simulink model "SimulinkNewUpdate"  (R2025a)
settings: Solver=VariableStepAuto  StartTime=0.0  StopTime=10.0  RelTol=1e-3
values from neighbouring files (symbols this model uses):
  AUM = 3.057    [Parameter.m]
  g = -9.8    [Parameter.m]
  H = 0.05    [Parameter.m]
  L = 0.25    [Parameter.m]
  rho = 1.18195    [Parameter.m]
  W = diag([0.994, 0.003, 0.003, 0.994, 0.003, 0.003,            0.994, 0.003, 0.003, 0.994, 0.003, 0.003])    [Parameter.m]
libraries: slpidlib x10, matrix_library x8, robotcorelib x4, simulink x1, uavalgslib x1, aerolibobsolete x1
(part 2 of 2)

== system SimulinkNewUpdate/Subsystem2/velocity control ==
  CmdvDown : Inport
  In Bus Element1 : Inport  Port=2  PortName=sensor
  In Bus Element : Inport  Port=2  PortName=sensor  Element=vZBody
  Discrete PID Controller : slpidlib/PID Controller  Controller=PID  Form=Parallel  TimeDomain=Discrete-time  UseExternalTs=off  SampleTime=0.005  IntegratorMethod=Forward Euler  FilterMethod=Forward Euler  ControllerParametersSource=external  P=1  I=1  UseKiTs=off  D=0  UseExternalDerivativeSource=off  N=100  UseFilter=on  TunerSelectOption=Transfer Function Based (PID Tuner App)  InitialConditionSource=external  InitialConditionForIntegrator=0  InitialConditionForFilter=0  DifferentiatorICPrevScaledInput=0  ExternalReset=none  TrackingMode=off  Kt=1  LimitOutput=on  SatLimitsSource=internal  UpperSaturationLimit=inf  LowerSaturationLimit=-inf  LinearizeAsGain=off  AntiWindupMode=none  Kb=1  LimitIntegrator=off  UpperIntegratorSaturationLimit=inf  LowerIntegratorSaturationLimit=-inf  POutMin=[]  POutMax=[]  IOutMin=[]  IOutMax=[]  DOutMin=[]  DOutMax=[]  NOutMin=[]  NOutMax=[]  SumOutMin=[]  SumOutMax=[]  SaturationOutMin=[]  SaturationOutMax=[]  PParamMin=[]  PParamMax=[]  IParamMin=[]  IParamMax=[]  DParamMin=[]  DParamMax=[]  NParamMin=[]  NParamMax=[]  KbParamMin=[]  KbParamMax=[]  KtParamMin=[]  KtParamMax=[]  KbOutMin=[]  KbOutMax=[]  KtOutMin=[]  KtOutMax=[]  IntegratorOutMin=[]  IntegratorOutMax=[]  FilterOutMin=[]  FilterOutMax=[]  SumI1OutMin=[]  SumI1OutMax=[]  SumI2OutMin=[]  SumI2OutMax=[]  SumI3OutMin=[]  SumI3OutMax=[]  SumI4OutMin=[]  SumI4OutMax=[]  SumDOutMin=[]  SumDOutMax=[]  DifferentiatorOutMin=[]  DifferentiatorOutMax=[]  FilterDiffOutCoefMin=[]  FilterDiffOutCoefMax=[]  ReciprocalOutMin=[]  ReciprocalOutMax=[]  SumDenOutMin=[]  SumDenOutMax=[]  SumNumOutMin=[]  SumNumOutMax=[]  DivideOutMin=[]  DivideOutMax=[]  UdiffTsProdOutMin=[]  UdiffTsProdOutMax=[]  NTsProdOutMin=[]  NTsProdOutMax=[]  UintegralTsProdOutMin=[]  UintegralTsProdOutMax=[]  UngainTsProdOutMin=[]  UngainTsProdOutMax=[]  ClampingZeroOutDataTypeStr=Inherit: Inherit via back propagation  ClampingZeroOutMin=[]  ClampingZeroOutMax=[]  FilterDenConstantOutDataTypeStr=Inherit: Inherit via back propagation  FilterDenConstantOutMin=[]  FilterDenConstantOutMax=[]  PCopyOutDataTypeStr=Inherit: Inherit via back propagation  PCopyOutMin=[]  PCopyOutMax=[]  NCopyOutDataTypeStr=Inherit: Inherit via back propagation  NCopyOutMin=[]  NCopyOutMax=[]  IntegratorContinuousStateAttributes=''  IntegratorStateMustResolveToSignalObject=off  IntegratorRTWStateStorageClass=Auto  FilterContinuousStateAttributes=''  FilterStateMustResolveToSignalObject=off  FilterRTWStateStorageClass=Auto  ParallelPVariant=ExternalParameters  IdealPVariant=Disabled  IVariant=ExternalParameters  DVariant=ExternalParameters  IntegratorVariant=Discrete  SatVariant=Enabled  AWVariant=Passthrough  PCopyVariant=Disabled  TRVariant=Disabled  FdbkBlocksVariant=Forward  IdealPFdbkVariant=Disabled  SatFdbkVariant=Disabled  DerivativeFilterVariant=ForwardEulerFilter  NVariant=ExternalParameters  NCopyVariant=Disabled  FilterICVariant=ExternalICs  IntegratorICVariant=ExternalICs  ExternalResetVariant=Disabled  TRSumVariant=Passthrough  SumFdbkVariant=Disabled  SumVariant=Sum_PID  TsampFilterVariant=InternalTs  TsampNgainVariant=Passthrough  TsampIntegralVariant=Disabled_SignalSpec  ExternalSaturationOutDataTypeStr=Inherit: Same as second input  DerivativeSourceVariant=ErrorSignal  PreIntVariant=InternalPreInt
      settings: LibrarySourceBlock=simulink/Discrete/Discrete PID Controller
  Gain : Gain  Gain=1000
  Kd : Constant
  Ki : Constant
  Kp : Constant
  N : Constant
  N1 : Constant
  N2 : Constant
  Roll and Pitch compensation : Subsystem
  Sum : Sum  Inputs=|+-
  cmdThrust : Outport
  wires:
  CmdvDown/1 -> Sum/1
  Sum/1 -> Discrete PID Controller/1
  Kp/1 -> Discrete PID Controller/2
  Ki/1 -> Discrete PID Controller/3
  Kd/1 -> Discrete PID Controller/4
  N/1 -> Discrete PID Controller/5
  Discrete PID Controller/1 -> Gain/1
  N1/1 -> Discrete PID Controller/6
  N2/1 -> Discrete PID Controller/7
  Gain/1 -> Roll and Pitch compensation/1(thrust)
  Roll and Pitch compensation/1(thrustCompensation) -> cmdThrust/1
  In Bus Element1/1 -> Roll and Pitch compensation/2(sensing)
  In Bus Element/1 -> Sum/2

== system SimulinkNewUpdate/Vehicle Dynamic1/Subsystem1 ==
  omega : Inport
  Bus Creator : BusCreator  Inputs=3
  Demux : Demux  Outputs=3
  Rotation : Outport
  wires:
  omega/1 -> Demux/1
  Bus Creator/1 -> Rotation/1
  Demux/1 -> Bus Creator/1  "p"
  Demux/2 -> Bus Creator/2  "q"
  Demux/3 -> Bus Creator/3  "r"

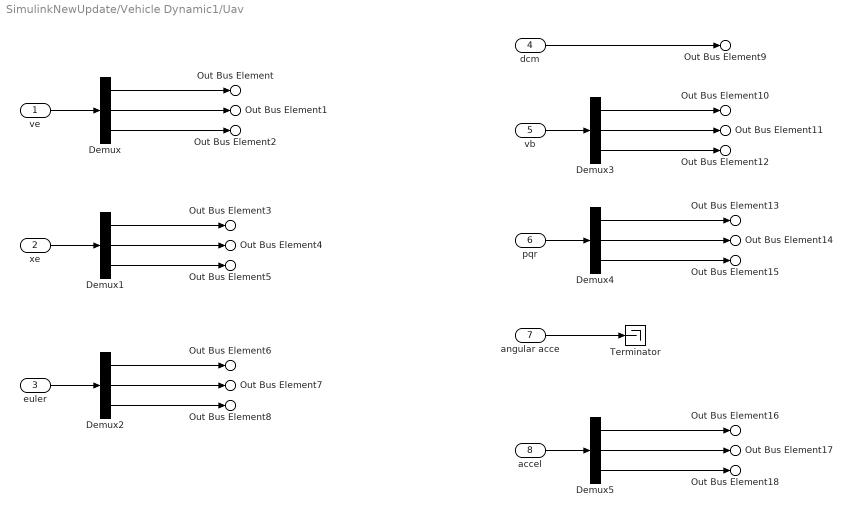
== system SimulinkNewUpdate/Vehicle Dynamic1/Uav ==
  ve : Inport
  xe : Inport  Port=2
  euler : Inport  Port=3
  dcm : Inport  Port=4
  vb : Inport  Port=5
  pqr : Inport  Port=6
  angular acce : Inport  Port=7
  accel : Inport  Port=8
  Demux{,1..5} (6 alike) : Demux  Outputs=3
  Terminator : Terminator
  Out Bus Element9 : Outport  PortName=UavState  Element=DCM
  Out Bus Element6 : Outport  PortName=UavState  Element=roll
  Out Bus Element7 : Outport  PortName=UavState  Element=pitch
  Out Bus Element8 : Outport  PortName=UavState  Element=yaw
  Out Bus Element : Outport  PortName=UavState  Element=veX
  Out Bus Element1 : Outport  PortName=UavState  Element=veY
  Out Bus Element2 : Outport  PortName=UavState  Element=veZ
  Out Bus Element3 : Outport  PortName=UavState  Element=x
  Out Bus Element4 : Outport  PortName=UavState  Element=y
  Out Bus Element5 : Outport  PortName=UavState  Element=z
  Out Bus Element10 : Outport  PortName=UavState  Element=vXBody
  Out Bus Element11 : Outport  PortName=UavState  Element=vYBody
  Out Bus Element12 : Outport  PortName=UavState  Element=vZBody
  Out Bus Element13 : Outport  PortName=UavState  Element=wx
  Out Bus Element14 : Outport  PortName=UavState  Element=wy
  Out Bus Element15 : Outport  PortName=UavState  Element=wz
  Out Bus Element16 : Outport  PortName=UavState  Element=accXBody
  Out Bus Element17 : Outport  PortName=UavState  Element=accYBody
  Out Bus Element18 : Outport  PortName=UavState  Element=accZBody
  wires:
  ve/1 -> Demux/1
  Demux/1 -> Out Bus Element/1
  Demux/2 -> Out Bus Element1/1
  Demux/3 -> Out Bus Element2/1
  xe/1 -> Demux1/1
  Demux1/1 -> Out Bus Element3/1
  Demux1/2 -> Out Bus Element4/1
  Demux1/3 -> Out Bus Element5/1
  euler/1 -> Demux2/1
  Demux2/1 -> Out Bus Element6/1
  Demux2/2 -> Out Bus Element7/1
  Demux2/3 -> Out Bus Element8/1
  dcm/1 -> Out Bus Element9/1
  vb/1 -> Demux3/1
  Demux3/1 -> Out Bus Element10/1
  Demux3/2 -> Out Bus Element11/1
  Demux3/3 -> Out Bus Element12/1
  pqr/1 -> Demux4/1
  Demux4/1 -> Out Bus Element13/1
  Demux4/2 -> Out Bus Element14/1
  Demux4/3 -> Out Bus Element15/1
  angular acce/1 -> Terminator/1
  accel/1 -> Demux5/1
  Demux5/1 -> Out Bus Element16/1
  Demux5/2 -> Out Bus Element17/1
  Demux5/3 -> Out Bus Element18/1

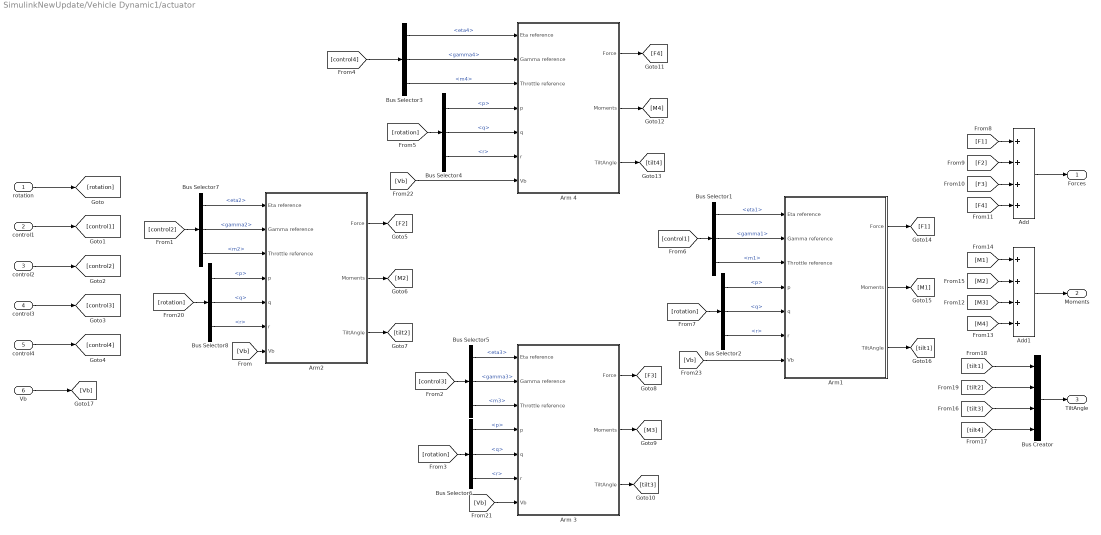
== system SimulinkNewUpdate/Vehicle Dynamic1/actuator ==
  rotation : Inport
  control1 : Inport  Port=2
  control2 : Inport  Port=3
  control3 : Inport  Port=4
  control4 : Inport  Port=5
  Vb : Inport  Port=6
  Add : Sum  Inputs=++++
  Add1 : Sum  Inputs=++++
  Arm 3 : Subsystem
  Arm 4 : Subsystem
  Arm1 : Subsystem
  Arm2 : Subsystem
  Bus Creator : BusCreator  Inputs=4
  Bus Selector1 : BusSelector  OutputSignals=eta1,gamma1,m1
  Bus Selector{2,4,6,8} (4 alike) : BusSelector  OutputSignals=p,q,r
  Bus Selector3 : BusSelector  OutputSignals=eta4,gamma4,m4
  Bus Selector5 : BusSelector  OutputSignals=eta3,gamma3,m3
  Bus Selector7 : BusSelector  OutputSignals=eta2,gamma2,m2
  Forces : Outport
  Moments : Outport  Port=2
  TiltAngle : Outport  Port=3
  wires:
  control3/1 -> [control3]
  Add/1 -> Forces/1
  [F4] -> Add/4
  [M3] -> Add1/3
  [control1] -> Bus Selector1/1
  Arm 4/1(Force) -> [F4]
  [M2] -> Add1/2
  Arm2/1(Force) -> [F2]
  [M1] -> Add1/1
  [M4] -> Add1/4
  Add1/1 -> Moments/1
  Arm 3/1(Force) -> [F3]
  Arm 4/2(Moments) -> [M4]
  Arm 3/2(Moments) -> [M3]
  control1/1 -> [control1]
  Arm2/3(TiltAngle) -> [tilt2]
  Arm 3/3(TiltAngle) -> [tilt3]
  control2/1 -> [control2]
  Arm2/2(Moments) -> [M2]
  Arm 4/3(TiltAngle) -> [tilt4]
  rotation/1 -> [rotation]
  control4/1 -> [control4]
  [F3] -> Add/3
  [F1] -> Add/1
  [F2] -> Add/2
  [tilt1] -> Bus Creator/1
  [tilt2] -> Bus Creator/2
  [tilt3] -> Bus Creator/3
  [tilt4] -> Bus Creator/4
  Bus Creator/1 -> TiltAngle/1
  [rotation] -> Bus Selector2/1
  Bus Selector1/1 -> Arm1/1(Eta reference)  "<eta1>"
  Bus Selector1/2 -> Arm1/2(Gamma reference)  "<gamma1>"
  Bus Selector1/3 -> Arm1/3(Throttle reference)  "<m1>"
  [control4] -> Bus Selector3/1
  [control3] -> Bus Selector5/1
  [control2] -> Bus Selector7/1
  Bus Selector5/1 -> Arm 3/1(Eta reference)  "<eta3>"
  Bus Selector5/2 -> Arm 3/2(Gamma reference)  "<gamma3>"
  Bus Selector5/3 -> Arm 3/3(Throttle reference)  "<m3>"
  Bus Selector7/1 -> Arm2/1(Eta reference)  "<eta2>"
  Bus Selector7/2 -> Arm2/2(Gamma reference)  "<gamma2>"
  Bus Selector7/3 -> Arm2/3(Throttle reference)  "<m2>"
  Bus Selector6/1 -> Arm 3/4(p)  "<p>"
  [rotation] -> Bus Selector6/1
  [rotation] -> Bus Selector8/1
  [rotation] -> Bus Selector4/1
  Bus Selector6/2 -> Arm 3/5(q)  "<q>"
  Bus Selector6/3 -> Arm 3/6(r)  "<r>"
  Arm1/1(Force) -> [F1]
  Arm1/2(Moments) -> [M1]
  Arm1/3(TiltAngle) -> [tilt1]
  Bus Selector2/1 -> Arm1/4(p)  "<p>"
  Bus Selector2/2 -> Arm1/5(q)  "<q>"
  Bus Selector2/3 -> Arm1/6(r)  "<r>"
  Bus Selector8/1 -> Arm2/4(p)  "<p>"
  Bus Selector8/2 -> Arm2/5(q)  "<q>"
  Bus Selector8/3 -> Arm2/6(r)  "<r>"
  Bus Selector3/1 -> Arm 4/1(Eta reference)  "<eta4>"
  Bus Selector3/2 -> Arm 4/2(Gamma reference)  "<gamma4>"
  Bus Selector3/3 -> Arm 4/3(Throttle reference)  "<m4>"
  Bus Selector4/1 -> Arm 4/4(p)  "<p>"
  Bus Selector4/2 -> Arm 4/5(q)  "<q>"
  Bus Selector4/3 -> Arm 4/6(r)  "<r>"
  Vb/1 -> [Vb]
  [Vb] -> Arm2/7(Vb)
  [Vb] -> Arm 3/7(Vb)
  [Vb] -> Arm 4/7(Vb)
  [Vb] -> Arm1/7(Vb)

== system SimulinkNewUpdate/Subsystem2/Subsystem/Subsystem ==
  yb_error : Inport
  vb_y : Inport  Port=2
  Pitch : Inport  Port=3
  Out1 : Outport
  wires:
  yb_error/1 -> Out1/1

== system SimulinkNewUpdate/Subsystem2/velocity control/Roll and Pitch compensation ==
  thrust : Inport
  In Bus Element : Inport  Port=2  PortName=sensing  Element=roll
  In Bus Element1 : Inport  Port=2  PortName=sensing  Element=pitch
  Constant : Constant
  Divide : Product  Inputs=*/
  Product : Product
  Product1 : Product
  Trigonometric Function : Trigonometry  Operator=cos
  Trigonometric Function1 : Trigonometry  Operator=cos
  "[0.5 ; 1]" : Saturate  UpperLimit=1  LowerLimit=0.5
  thrustCompensation : Outport
  wires:
  thrust/1 -> Product1/1
  Trigonometric Function1/1 -> Product/2
  Trigonometric Function/1 -> Product/1
  Product/1 -> "[0.5 ; 1]"/1
  "[0.5 ; 1]"/1 -> Divide/2
  Constant/1 -> Divide/1
  Divide/1 -> Product1/2
  Product1/1 -> thrustCompensation/1
  In Bus Element1/1 -> Trigonometric Function1/1
  In Bus Element/1 -> Trigonometric Function/1

== system SimulinkNewUpdate/Vehicle Dynamic1/actuator/Arm 3 ==
  Eta reference : Inport
  Gamma reference : Inport  Port=2
  Throttle reference : Inport  Port=3
  p : Inport  Port=4
  q : Inport  Port=5
  r : Inport  Port=6
  Vb : Inport  Port=7
  Constant : Constant  Value=[1 0 0; 0 1 0; 0 0 1]
  Constant1 : Constant
  Matrix Multiply : Product  Multiplication=Matrix(*)
  Matrix Multiply1 : Product  Multiplication=Matrix(*)
  STANDARD ARM MODEL CLOCKWISE : Subsystem
  Force : Outport
  Moments : Outport  Port=2
  TiltAngle : Outport  Port=3
  wires:
  Gamma reference/1 -> STANDARD ARM MODEL CLOCKWISE/2(Gamma reference)
  Eta reference/1 -> STANDARD ARM MODEL CLOCKWISE/1(Eta reference)
  Matrix Multiply1/1 -> Moments/1
  STANDARD ARM MODEL CLOCKWISE/1(F) -> Matrix Multiply/2
  Throttle reference/1 -> STANDARD ARM MODEL CLOCKWISE/3(Throttle reference)
  r/1 -> STANDARD ARM MODEL CLOCKWISE/6(r)
  p/1 -> STANDARD ARM MODEL CLOCKWISE/4(p)
  q/1 -> STANDARD ARM MODEL CLOCKWISE/5(q)
  STANDARD ARM MODEL CLOCKWISE/2(M) -> Matrix Multiply1/2
  Constant/1 -> Matrix Multiply1/1, Matrix Multiply/1
  Matrix Multiply/1 -> Force/1
  STANDARD ARM MODEL CLOCKWISE/3(TiltAngle) -> TiltAngle/1
  Vb/1 -> STANDARD ARM MODEL CLOCKWISE/7(Vb)
  Constant1/1 -> STANDARD ARM MODEL CLOCKWISE/8(TurnDirection)

== system SimulinkNewUpdate/Vehicle Dynamic1/actuator/Arm 4 ==
  Eta reference : Inport
  Gamma reference : Inport  Port=2
  Throttle reference : Inport  Port=3
  p : Inport  Port=4
  q : Inport  Port=5
  r : Inport  Port=6
  Vb : Inport  Port=7
  Constant : Constant  Value=[-1 0 0;0 -1 0; 0 0 1]
  Constant2 : Constant
  Matrix Multiply : Product  Multiplication=Matrix(*)
  Matrix Multiply1 : Product  Multiplication=Matrix(*)
  STANDARD ARM MODEL CLOCKWISE : Subsystem
  Force : Outport
  Moments : Outport  Port=2
  TiltAngle : Outport  Port=3
  wires:
  Vb/1 -> STANDARD ARM MODEL CLOCKWISE/7(Vb)
  Constant2/1 -> STANDARD ARM MODEL CLOCKWISE/8(TurnDirection)
  Matrix Multiply1/1 -> Moments/1
  Matrix Multiply/1 -> Force/1
  STANDARD ARM MODEL CLOCKWISE/3(TiltAngle) -> TiltAngle/1
  p/1 -> STANDARD ARM MODEL CLOCKWISE/4(p)
  Eta reference/1 -> STANDARD ARM MODEL CLOCKWISE/1(Eta reference)
  r/1 -> STANDARD ARM MODEL CLOCKWISE/6(r)
  STANDARD ARM MODEL CLOCKWISE/1(F) -> Matrix Multiply/2
  STANDARD ARM MODEL CLOCKWISE/2(M) -> Matrix Multiply1/2
  Constant/1 -> Matrix Multiply1/1, Matrix Multiply/1
  q/1 -> STANDARD ARM MODEL CLOCKWISE/5(q)
  Gamma reference/1 -> STANDARD ARM MODEL CLOCKWISE/2(Gamma reference)
  Throttle reference/1 -> STANDARD ARM MODEL CLOCKWISE/3(Throttle reference)

== system SimulinkNewUpdate/Vehicle Dynamic1/actuator/Arm1 ==
  Eta reference : Inport
  Gamma reference : Inport  Port=2
  Throttle reference : Inport  Port=3
  p : Inport  Port=4
  q : Inport  Port=5
  r : Inport  Port=6
  Vb : Inport  Port=7
  Constant : Constant  Value=[0 1 0; -1 0 0; 0 0 1]
  Constant2 : Constant  Value=-1
  Matrix Multiply : Product  Multiplication=Matrix(*)
  Matrix Multiply1 : Product  Multiplication=Matrix(*)
  STANDARD ARM MODEL CLOCKWISE : Subsystem
  Force : Outport
  Moments : Outport  Port=2
  TiltAngle : Outport  Port=3
  wires:
  Vb/1 -> STANDARD ARM MODEL CLOCKWISE/7(Vb)
  Constant2/1 -> STANDARD ARM MODEL CLOCKWISE/8(TurnDirection)
  Matrix Multiply1/1 -> Moments/1
  Matrix Multiply/1 -> Force/1
  STANDARD ARM MODEL CLOCKWISE/3(TiltAngle) -> TiltAngle/1
  p/1 -> STANDARD ARM MODEL CLOCKWISE/4(p)
  Eta reference/1 -> STANDARD ARM MODEL CLOCKWISE/1(Eta reference)
  r/1 -> STANDARD ARM MODEL CLOCKWISE/6(r)
  STANDARD ARM MODEL CLOCKWISE/1(F) -> Matrix Multiply/2
  STANDARD ARM MODEL CLOCKWISE/2(M) -> Matrix Multiply1/2
  Constant/1 -> Matrix Multiply1/1, Matrix Multiply/1
  q/1 -> STANDARD ARM MODEL CLOCKWISE/5(q)
  Gamma reference/1 -> STANDARD ARM MODEL CLOCKWISE/2(Gamma reference)
  Throttle reference/1 -> STANDARD ARM MODEL CLOCKWISE/3(Throttle reference)

== system SimulinkNewUpdate/Vehicle Dynamic1/actuator/Arm2 ==
  Eta reference : Inport
  Gamma reference : Inport  Port=2
  Throttle reference : Inport  Port=3
  p : Inport  Port=4
  q : Inport  Port=5
  r : Inport  Port=6
  Vb : Inport  Port=7
  Constant : Constant  Value=[0 -1 0; 1 0 0; 0 0 1]
  Constant2 : Constant  Value=-1
  Matrix Multiply : Product  Multiplication=Matrix(*)
  Matrix Multiply1 : Product  Multiplication=Matrix(*)
  STANDARD ARM MODEL CLOCKWISE : Subsystem
  Force : Outport
  Moments : Outport  Port=2
  TiltAngle : Outport  Port=3
  wires:
  Vb/1 -> STANDARD ARM MODEL CLOCKWISE/7(Vb)
  Constant2/1 -> STANDARD ARM MODEL CLOCKWISE/8(TurnDirection)
  Matrix Multiply1/1 -> Moments/1
  Matrix Multiply/1 -> Force/1
  STANDARD ARM MODEL CLOCKWISE/3(TiltAngle) -> TiltAngle/1
  p/1 -> STANDARD ARM MODEL CLOCKWISE/4(p)
  Eta reference/1 -> STANDARD ARM MODEL CLOCKWISE/1(Eta reference)
  r/1 -> STANDARD ARM MODEL CLOCKWISE/6(r)
  STANDARD ARM MODEL CLOCKWISE/1(F) -> Matrix Multiply/2
  STANDARD ARM MODEL CLOCKWISE/2(M) -> Matrix Multiply1/2
  Constant/1 -> Matrix Multiply1/1, Matrix Multiply/1
  q/1 -> STANDARD ARM MODEL CLOCKWISE/5(q)
  Gamma reference/1 -> STANDARD ARM MODEL CLOCKWISE/2(Gamma reference)
  Throttle reference/1 -> STANDARD ARM MODEL CLOCKWISE/3(Throttle reference)

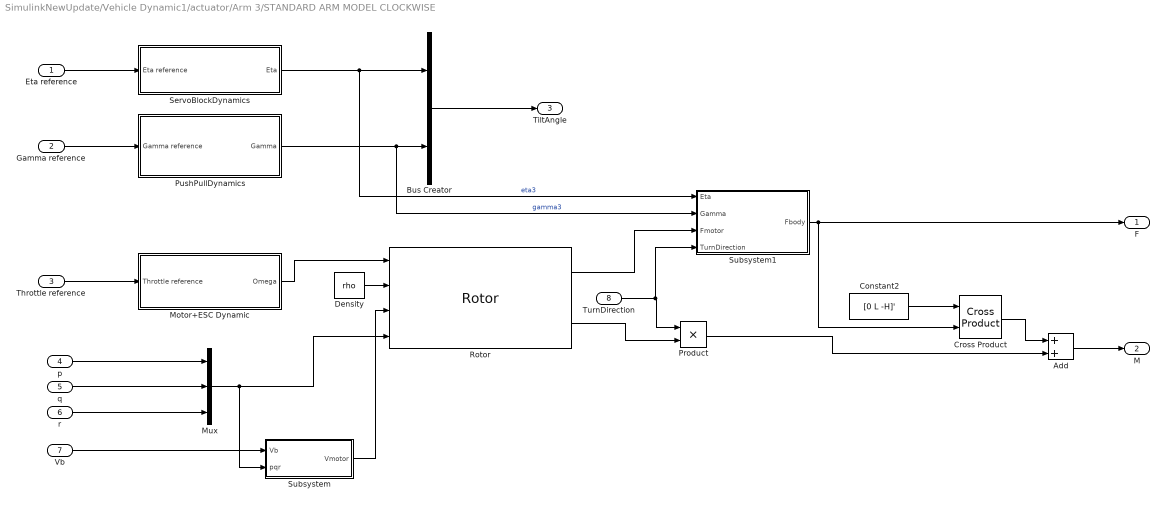
== system SimulinkNewUpdate/Vehicle Dynamic1/actuator/Arm 3/STANDARD ARM MODEL CLOCKWISE ==
  Eta reference : Inport
  Gamma reference : Inport  Port=2
  Throttle reference : Inport  Port=3
  p : Inport  Port=4
  q : Inport  Port=5
  r : Inport  Port=6
  Vb : Inport  Port=7
  TurnDirection : Inport  Port=8
  Add : Sum
  Bus Creator : BusCreator  Inputs=2
  Constant2 : Constant  Value=[0 L -H]'
  Cross Product : matrix_library/Cross Product
  Density : Constant  Value=rho
  Motor+ESC Dynamic : Subsystem
  Mux : Mux  Inputs=3
  Product : Product
  PushPullDynamics : Subsystem
  Rotor : Rotor  modelMode=With flap effects  CT=Ct  CQ=Cq  Nb=3  radius=0.1905
  ServoBlockDynamics : Subsystem
  Subsystem : Subsystem
  Subsystem1 : Subsystem
  F : Outport
  M : Outport  Port=2
  TiltAngle : Outport  Port=3
  wires:
  p/1 -> Mux/1
  Gamma reference/1 -> PushPullDynamics/1(Gamma reference)
  Throttle reference/1 -> Motor+ESC Dynamic/1(Throttle reference)
  q/1 -> Mux/2
  Density/1 -> Rotor/2
  Motor+ESC Dynamic/1(Omega) -> Rotor/1
  r/1 -> Mux/3
  Eta reference/1 -> ServoBlockDynamics/1(Eta reference)
  Bus Creator/1 -> TiltAngle/1
  PushPullDynamics/1(Gamma) -> Subsystem1/2(Gamma), Bus Creator/2  "gamma3"
  ServoBlockDynamics/1(Eta) -> Subsystem1/1(Eta), Bus Creator/1  "eta3"
  Mux/1 -> Subsystem/2(pqr), Rotor/4
  Vb/1 -> Subsystem/1(Vb)
  Subsystem/1(Vmotor) -> Rotor/3
  Rotor/1 -> Subsystem1/3(Fmotor)
  Rotor/2 -> Product/2
  TurnDirection/1 -> Subsystem1/4(TurnDirection), Product/1
  Subsystem1/1(Fbody) -> Cross Product/2, F/1
  Add/1 -> M/1
  Constant2/1 -> Cross Product/1
  Cross Product/1 -> Add/1
  Product/1 -> Add/2

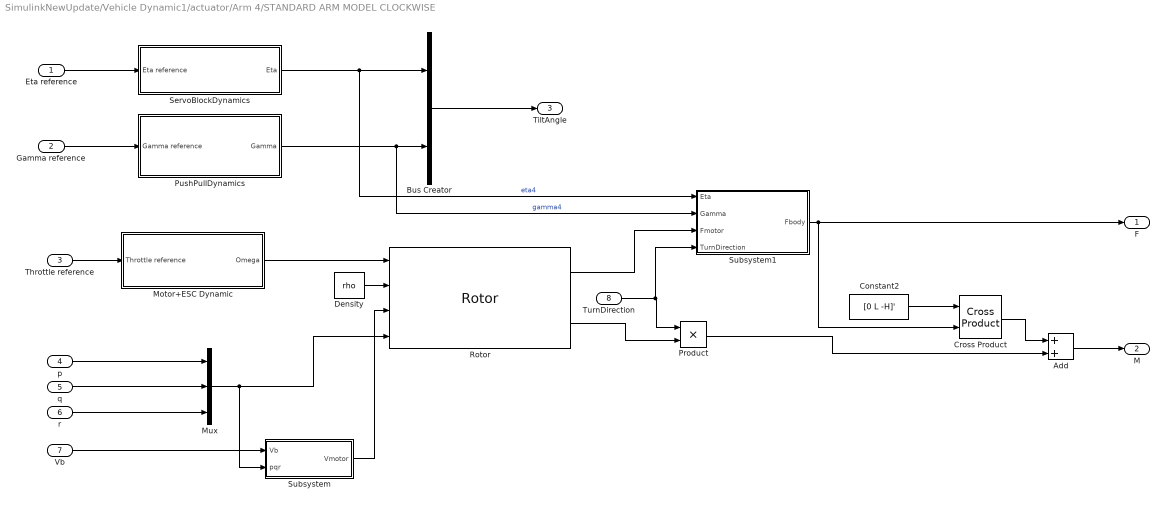
== system SimulinkNewUpdate/Vehicle Dynamic1/actuator/Arm 4/STANDARD ARM MODEL CLOCKWISE ==
  Eta reference : Inport
  Gamma reference : Inport  Port=2
  Throttle reference : Inport  Port=3
  p : Inport  Port=4
  q : Inport  Port=5
  r : Inport  Port=6
  Vb : Inport  Port=7
  TurnDirection : Inport  Port=8
  Add : Sum
  Bus Creator : BusCreator  Inputs=2
  Constant2 : Constant  Value=[0 L -H]'
  Cross Product : matrix_library/Cross Product
  Density : Constant  Value=rho
  Motor+ESC Dynamic : Subsystem
  Mux : Mux  Inputs=3
  Product : Product
  PushPullDynamics : Subsystem
  Rotor : Rotor  modelMode=With flap effects  CT=Ct  CQ=Cq  Nb=3  radius=0.1905
  ServoBlockDynamics : Subsystem
  Subsystem : Subsystem
  Subsystem1 : Subsystem
  F : Outport
  M : Outport  Port=2
  TiltAngle : Outport  Port=3
  wires:
  p/1 -> Mux/1
  Gamma reference/1 -> PushPullDynamics/1(Gamma reference)
  Throttle reference/1 -> Motor+ESC Dynamic/1(Throttle reference)
  q/1 -> Mux/2
  Density/1 -> Rotor/2
  Motor+ESC Dynamic/1(Omega) -> Rotor/1
  r/1 -> Mux/3
  Eta reference/1 -> ServoBlockDynamics/1(Eta reference)
  Bus Creator/1 -> TiltAngle/1
  PushPullDynamics/1(Gamma) -> Subsystem1/2(Gamma), Bus Creator/2  "gamma4"
  ServoBlockDynamics/1(Eta) -> Subsystem1/1(Eta), Bus Creator/1  "eta4"
  Mux/1 -> Subsystem/2(pqr), Rotor/4
  Vb/1 -> Subsystem/1(Vb)
  Subsystem/1(Vmotor) -> Rotor/3
  Rotor/1 -> Subsystem1/3(Fmotor)
  Rotor/2 -> Product/2
  TurnDirection/1 -> Subsystem1/4(TurnDirection), Product/1
  Subsystem1/1(Fbody) -> Cross Product/2, F/1
  Add/1 -> M/1
  Constant2/1 -> Cross Product/1
  Cross Product/1 -> Add/1
  Product/1 -> Add/2

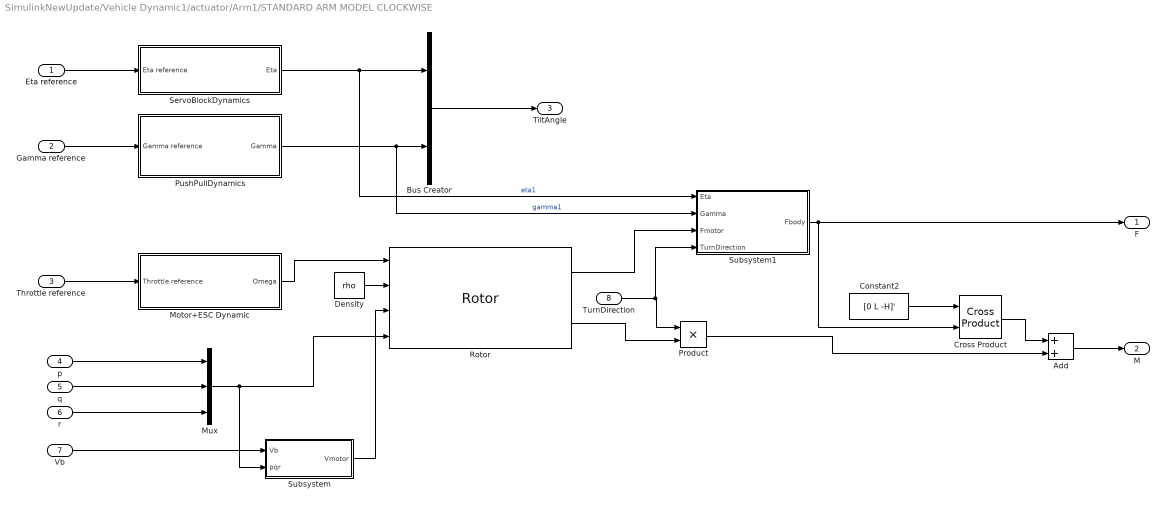
== system SimulinkNewUpdate/Vehicle Dynamic1/actuator/Arm1/STANDARD ARM MODEL CLOCKWISE ==
  Eta reference : Inport
  Gamma reference : Inport  Port=2
  Throttle reference : Inport  Port=3
  p : Inport  Port=4
  q : Inport  Port=5
  r : Inport  Port=6
  Vb : Inport  Port=7
  TurnDirection : Inport  Port=8
  Add : Sum
  Bus Creator : BusCreator  Inputs=2
  Constant2 : Constant  Value=[0 L -H]'
  Cross Product : matrix_library/Cross Product
  Density : Constant  Value=rho
  Motor+ESC Dynamic : Subsystem
  Mux : Mux  Inputs=3
  Product : Product
  PushPullDynamics : Subsystem
  Rotor : Rotor  modelMode=With flap effects  CT=Ct  CQ=Cq  Nb=3  radius=0.1905
  ServoBlockDynamics : Subsystem
  Subsystem : Subsystem
  Subsystem1 : Subsystem
  F : Outport
  M : Outport  Port=2
  TiltAngle : Outport  Port=3
  wires:
  p/1 -> Mux/1
  Gamma reference/1 -> PushPullDynamics/1(Gamma reference)
  Throttle reference/1 -> Motor+ESC Dynamic/1(Throttle reference)
  q/1 -> Mux/2
  Density/1 -> Rotor/2
  Motor+ESC Dynamic/1(Omega) -> Rotor/1
  r/1 -> Mux/3
  Eta reference/1 -> ServoBlockDynamics/1(Eta reference)
  Bus Creator/1 -> TiltAngle/1
  PushPullDynamics/1(Gamma) -> Subsystem1/2(Gamma), Bus Creator/2  "gamma1"
  ServoBlockDynamics/1(Eta) -> Subsystem1/1(Eta), Bus Creator/1  "eta1"
  Mux/1 -> Subsystem/2(pqr), Rotor/4
  Vb/1 -> Subsystem/1(Vb)
  Subsystem/1(Vmotor) -> Rotor/3
  Rotor/1 -> Subsystem1/3(Fmotor)
  Rotor/2 -> Product/2
  TurnDirection/1 -> Subsystem1/4(TurnDirection), Product/1
  Subsystem1/1(Fbody) -> Cross Product/2, F/1
  Add/1 -> M/1
  Constant2/1 -> Cross Product/1
  Cross Product/1 -> Add/1
  Product/1 -> Add/2

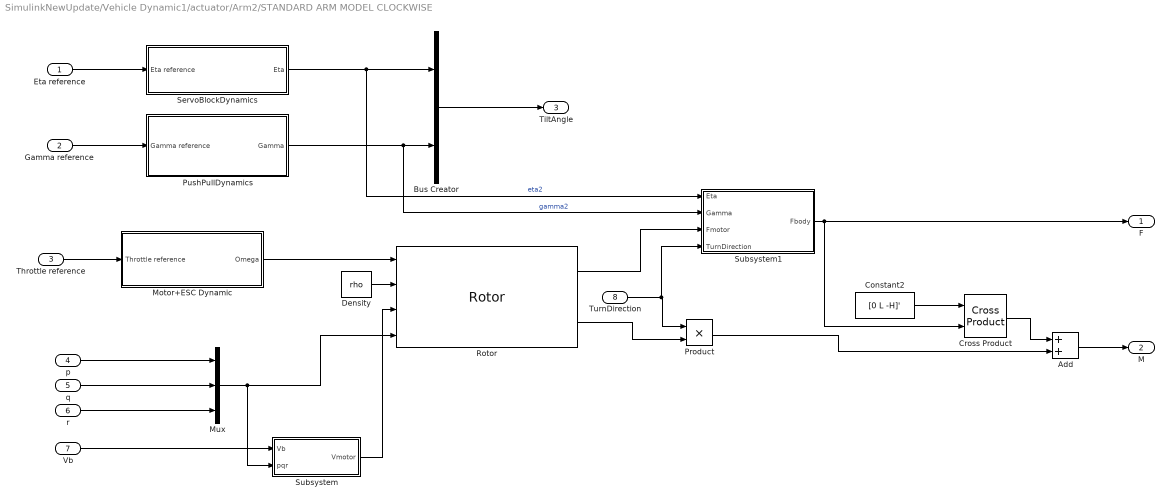
== system SimulinkNewUpdate/Vehicle Dynamic1/actuator/Arm2/STANDARD ARM MODEL CLOCKWISE ==
  Eta reference : Inport
  Gamma reference : Inport  Port=2
  Throttle reference : Inport  Port=3
  p : Inport  Port=4
  q : Inport  Port=5
  r : Inport  Port=6
  Vb : Inport  Port=7
  TurnDirection : Inport  Port=8
  Add : Sum
  Bus Creator : BusCreator  Inputs=2
  Constant2 : Constant  Value=[0 L -H]'
  Cross Product : matrix_library/Cross Product
  Density : Constant  Value=rho
  Motor+ESC Dynamic : Subsystem
  Mux : Mux  Inputs=3
  Product : Product
  PushPullDynamics : Subsystem
  Rotor : Rotor  modelMode=With flap effects  CT=Ct  CQ=Cq  Nb=3  radius=0.1905
  ServoBlockDynamics : Subsystem
  Subsystem : Subsystem
  Subsystem1 : Subsystem
  F : Outport
  M : Outport  Port=2
  TiltAngle : Outport  Port=3
  wires:
  p/1 -> Mux/1
  Gamma reference/1 -> PushPullDynamics/1(Gamma reference)
  Throttle reference/1 -> Motor+ESC Dynamic/1(Throttle reference)
  q/1 -> Mux/2
  Density/1 -> Rotor/2
  Motor+ESC Dynamic/1(Omega) -> Rotor/1
  r/1 -> Mux/3
  Eta reference/1 -> ServoBlockDynamics/1(Eta reference)
  Bus Creator/1 -> TiltAngle/1
  PushPullDynamics/1(Gamma) -> Subsystem1/2(Gamma), Bus Creator/2  "gamma2"
  ServoBlockDynamics/1(Eta) -> Subsystem1/1(Eta), Bus Creator/1  "eta2"
  Mux/1 -> Subsystem/2(pqr), Rotor/4
  Vb/1 -> Subsystem/1(Vb)
  Subsystem/1(Vmotor) -> Rotor/3
  Rotor/1 -> Subsystem1/3(Fmotor)
  Rotor/2 -> Product/2
  TurnDirection/1 -> Subsystem1/4(TurnDirection), Product/1
  Subsystem1/1(Fbody) -> Cross Product/2, F/1
  Add/1 -> M/1
  Constant2/1 -> Cross Product/1
  Cross Product/1 -> Add/1
  Product/1 -> Add/2

== system SimulinkNewUpdate/Vehicle Dynamic1/actuator/Arm 3/STANDARD ARM MODEL CLOCKWISE/Motor+ESC Dynamic ==
  Throttle reference : Inport
  G Motor : TransferFcn  Numerator=[9.19]  Denominator=[0.16 1]
  Gain : Gain  Gain=2*pi/60
  Saturation : Saturate  UpperLimit=7685  LowerLimit=0
  Omega : Outport
  wires:
  Throttle reference/1 -> G Motor/1
  G Motor/1 -> Saturation/1
  Gain/1 -> Omega/1
  Saturation/1 -> Gain/1

== system SimulinkNewUpdate/Vehicle Dynamic1/actuator/Arm 3/STANDARD ARM MODEL CLOCKWISE/PushPullDynamics ==
  Gamma reference : Inport
  G pushpull : TransferFcn  Numerator=[1212.73]  Denominator=[1 51.105 1212.73]
  Saturation : Saturate  UpperLimit=pi/9  LowerLimit=-pi/9
  Saturation1 : Saturate  UpperLimit=pi/9  LowerLimit=-pi/9
  Gamma : Outport
  wires:
  Gamma reference/1 -> Saturation/1
  G pushpull/1 -> Saturation1/1
  Saturation/1 -> G pushpull/1
  Saturation1/1 -> Gamma/1

== system SimulinkNewUpdate/Vehicle Dynamic1/actuator/Arm 3/STANDARD ARM MODEL CLOCKWISE/ServoBlockDynamics ==
  Eta reference : Inport
  G Servoblock : TransferFcn  Numerator=[1228.05]  Denominator=[1 49.1806 1228.05]
  Saturation : Saturate  UpperLimit=pi/9  LowerLimit=-pi/9
  Saturation1 : Saturate  UpperLimit=pi/9  LowerLimit=-pi/9
  Eta : Outport
  wires:
  Eta reference/1 -> Saturation/1
  G Servoblock/1 -> Saturation1/1
  Saturation/1 -> G Servoblock/1
  Saturation1/1 -> Eta/1

== system SimulinkNewUpdate/Vehicle Dynamic1/actuator/Arm 3/STANDARD ARM MODEL CLOCKWISE/Subsystem ==
  Vb : Inport
  pqr : Inport  Port=2
  Add : Sum
  Constant2 : Constant  Value=[0 L H]'
  Cross Product : matrix_library/Cross Product
  Reshape : Reshape  OutputDimensionality=Column vector (2-D)
  Vmotor : Outport
  wires:
  Vb/1 -> Reshape/1
  Constant2/1 -> Cross Product/1
  pqr/1 -> Cross Product/2
  Reshape/1 -> Add/1
  Cross Product/1 -> Add/2
  Add/1 -> Vmotor/1

== system SimulinkNewUpdate/Vehicle Dynamic1/actuator/Arm 3/STANDARD ARM MODEL CLOCKWISE/Subsystem1 ==
  Eta : Inport
  Gamma : Inport  Port=2
  Fmotor : Inport  Port=3
  TurnDirection : Inport  Port=4
  Constant : Constant  Value=0
  Constant1 : Constant
  Constant3 : Constant
  Coordinate Transformation Conversion : robotcorelib/Coordinate Transformation Conversion  InputRepresentation=Euler Angles  InputEulerSequence=ZYX  ShowTrVecInputPort=on  OutputRepresentation=Rotation Matrix  OutputEulerSequence=ZYX  ShowTrVecOutputPort=on  SimulateUsing=Interpreted execution
      settings: LibrarySourceBlock=uavutilslib/Coordinate Transformation Conversion
  Gain1 : Gain  Gain=-1
  Gain2 : Gain  Gain=-1
  MatrixMultiply : Product  Multiplication=Matrix(*)
  Mux : Mux  Inputs=3
  Mux1 : Mux  Inputs=3
  Product : Product
  Fbody : Outport
  wires:
  Constant/1 -> Mux/1
  Eta/1 -> Gain1/1
  Gamma/1 -> Gain2/1
  Mux/1 -> Coordinate Transformation Conversion/1
  Constant1/1 -> Mux1/1
  TurnDirection/1 -> Mux1/2
  Constant3/1 -> Mux1/3
  Fmotor/1 -> Product/1
  Mux1/1 -> Product/2
  Coordinate Transformation Conversion/1 -> MatrixMultiply/1
  Product/1 -> MatrixMultiply/2
  MatrixMultiply/1 -> Fbody/1
  Gain2/1 -> Mux/3
  Gain1/1 -> Mux/2

== system SimulinkNewUpdate/Vehicle Dynamic1/actuator/Arm 4/STANDARD ARM MODEL CLOCKWISE/Motor+ESC Dynamic ==
  Throttle reference : Inport
  G Motor : TransferFcn  Numerator=[9.19]  Denominator=[0.16 1]
  Gain : Gain  Gain=2*pi/60
  Saturation : Saturate  UpperLimit=7685  LowerLimit=0
  Omega : Outport
  wires:
  Throttle reference/1 -> G Motor/1
  G Motor/1 -> Saturation/1
  Gain/1 -> Omega/1
  Saturation/1 -> Gain/1

== system SimulinkNewUpdate/Vehicle Dynamic1/actuator/Arm 4/STANDARD ARM MODEL CLOCKWISE/PushPullDynamics ==
  Gamma reference : Inport
  G pushpull : TransferFcn  Numerator=[1212.73]  Denominator=[1 51.105 1212.73]
  Saturation : Saturate  UpperLimit=pi/9  LowerLimit=-pi/9
  Saturation1 : Saturate  UpperLimit=pi/9  LowerLimit=-pi/9
  Gamma : Outport
  wires:
  Gamma reference/1 -> Saturation/1
  G pushpull/1 -> Saturation1/1
  Saturation/1 -> G pushpull/1
  Saturation1/1 -> Gamma/1

== system SimulinkNewUpdate/Vehicle Dynamic1/actuator/Arm 4/STANDARD ARM MODEL CLOCKWISE/ServoBlockDynamics ==
  Eta reference : Inport
  G Servoblock : TransferFcn  Numerator=[1228.05]  Denominator=[1 49.1806 1228.05]
  Saturation : Saturate  UpperLimit=pi/9  LowerLimit=-pi/9
  Saturation1 : Saturate  UpperLimit=pi/9  LowerLimit=-pi/9
  Eta : Outport
  wires:
  Eta reference/1 -> Saturation/1
  G Servoblock/1 -> Saturation1/1
  Saturation/1 -> G Servoblock/1
  Saturation1/1 -> Eta/1

== system SimulinkNewUpdate/Vehicle Dynamic1/actuator/Arm 4/STANDARD ARM MODEL CLOCKWISE/Subsystem ==
  Vb : Inport
  pqr : Inport  Port=2
  Add : Sum
  Constant2 : Constant  Value=[0 L H]'
  Cross Product : matrix_library/Cross Product
  Reshape : Reshape  OutputDimensionality=Column vector (2-D)
  Vmotor : Outport
  wires:
  Vb/1 -> Reshape/1
  Constant2/1 -> Cross Product/1
  pqr/1 -> Cross Product/2
  Reshape/1 -> Add/1
  Cross Product/1 -> Add/2
  Add/1 -> Vmotor/1

== system SimulinkNewUpdate/Vehicle Dynamic1/actuator/Arm 4/STANDARD ARM MODEL CLOCKWISE/Subsystem1 ==
  Eta : Inport
  Gamma : Inport  Port=2
  Fmotor : Inport  Port=3
  TurnDirection : Inport  Port=4
  Constant : Constant  Value=0
  Constant1 : Constant
  Constant3 : Constant
  Coordinate Transformation Conversion : robotcorelib/Coordinate Transformation Conversion  InputRepresentation=Euler Angles  InputEulerSequence=ZYX  ShowTrVecInputPort=on  OutputRepresentation=Rotation Matrix  OutputEulerSequence=ZYX  ShowTrVecOutputPort=on  SimulateUsing=Interpreted execution
      settings: LibrarySourceBlock=uavutilslib/Coordinate Transformation Conversion
  Gain : Gain  Gain=-1
  Gain1 : Gain  Gain=-1
  MatrixMultiply : Product  Multiplication=Matrix(*)
  Mux : Mux  Inputs=3
  Mux1 : Mux  Inputs=3
  Product : Product
  Fbody : Outport
  wires:
  Constant/1 -> Mux/1
  Eta/1 -> Gain/1
  Gamma/1 -> Gain1/1
  Mux/1 -> Coordinate Transformation Conversion/1
  Constant1/1 -> Mux1/1
  TurnDirection/1 -> Mux1/2
  Constant3/1 -> Mux1/3
  Fmotor/1 -> Product/1
  Mux1/1 -> Product/2
  Coordinate Transformation Conversion/1 -> MatrixMultiply/1
  Product/1 -> MatrixMultiply/2
  MatrixMultiply/1 -> Fbody/1
  Gain/1 -> Mux/2
  Gain1/1 -> Mux/3

== system SimulinkNewUpdate/Vehicle Dynamic1/actuator/Arm1/STANDARD ARM MODEL CLOCKWISE/Motor+ESC Dynamic ==
  Throttle reference : Inport
  G Motor : TransferFcn  Numerator=[9.19]  Denominator=[0.16 1]
  Gain : Gain  Gain=2*pi/60
  Saturation : Saturate  UpperLimit=7685  LowerLimit=0
  Omega : Outport
  wires:
  Throttle reference/1 -> G Motor/1
  G Motor/1 -> Saturation/1
  Gain/1 -> Omega/1
  Saturation/1 -> Gain/1

== system SimulinkNewUpdate/Vehicle Dynamic1/actuator/Arm1/STANDARD ARM MODEL CLOCKWISE/PushPullDynamics ==
  Gamma reference : Inport
  G pushpull : TransferFcn  Numerator=[1212.73]  Denominator=[1 51.105 1212.73]
  Saturation : Saturate  UpperLimit=pi/9  LowerLimit=-pi/9
  Saturation1 : Saturate  UpperLimit=pi/9  LowerLimit=-pi/9
  Gamma : Outport
  wires:
  Gamma reference/1 -> Saturation/1
  G pushpull/1 -> Saturation1/1
  Saturation/1 -> G pushpull/1
  Saturation1/1 -> Gamma/1

== system SimulinkNewUpdate/Vehicle Dynamic1/actuator/Arm1/STANDARD ARM MODEL CLOCKWISE/ServoBlockDynamics ==
  Eta reference : Inport
  G Servoblock : TransferFcn  Numerator=[1228.05]  Denominator=[1 49.1806 1228.05]
  Saturation : Saturate  UpperLimit=pi/9  LowerLimit=-pi/9
  Saturation1 : Saturate  UpperLimit=pi/9  LowerLimit=-pi/9
  Eta : Outport
  wires:
  Eta reference/1 -> Saturation/1
  G Servoblock/1 -> Saturation1/1
  Saturation/1 -> G Servoblock/1
  Saturation1/1 -> Eta/1

== system SimulinkNewUpdate/Vehicle Dynamic1/actuator/Arm1/STANDARD ARM MODEL CLOCKWISE/Subsystem ==
  Vb : Inport
  pqr : Inport  Port=2
  Add : Sum
  Constant2 : Constant  Value=[0 L H]'
  Cross Product : matrix_library/Cross Product
  Reshape : Reshape  OutputDimensionality=Column vector (2-D)
  Vmotor : Outport
  wires:
  Vb/1 -> Reshape/1
  Constant2/1 -> Cross Product/1
  pqr/1 -> Cross Product/2
  Reshape/1 -> Add/1
  Cross Product/1 -> Add/2
  Add/1 -> Vmotor/1

== system SimulinkNewUpdate/Vehicle Dynamic1/actuator/Arm1/STANDARD ARM MODEL CLOCKWISE/Subsystem1 ==
  Eta : Inport
  Gamma : Inport  Port=2
  Fmotor : Inport  Port=3
  TurnDirection : Inport  Port=4
  Constant : Constant  Value=0
  Constant1 : Constant
  Constant3 : Constant
  Coordinate Transformation Conversion : robotcorelib/Coordinate Transformation Conversion  InputRepresentation=Euler Angles  InputEulerSequence=ZYX  ShowTrVecInputPort=on  OutputRepresentation=Rotation Matrix  OutputEulerSequence=ZYX  ShowTrVecOutputPort=on  SimulateUsing=Interpreted execution
      settings: LibrarySourceBlock=uavutilslib/Coordinate Transformation Conversion
  Gain1 : Gain  Gain=-1
  Gain2 : Gain  Gain=-1
  Gain3 : Gain  Gain=-1
  MatrixMultiply : Product  Multiplication=Matrix(*)
  Mux : Mux  Inputs=3
  Mux1 : Mux  Inputs=3
  Product : Product
  Fbody : Outport
  wires:
  Constant/1 -> Gain1/1
  Eta/1 -> Gain2/1
  Gamma/1 -> Gain3/1
  Mux/1 -> Coordinate Transformation Conversion/1
  Constant1/1 -> Mux1/1
  TurnDirection/1 -> Mux1/2
  Constant3/1 -> Mux1/3
  Fmotor/1 -> Product/1
  Mux1/1 -> Product/2
  Coordinate Transformation Conversion/1 -> MatrixMultiply/1
  Product/1 -> MatrixMultiply/2
  MatrixMultiply/1 -> Fbody/1
  Gain1/1 -> Mux/1
  Gain2/1 -> Mux/2
  Gain3/1 -> Mux/3

== system SimulinkNewUpdate/Vehicle Dynamic1/actuator/Arm2/STANDARD ARM MODEL CLOCKWISE/Motor+ESC Dynamic ==
  Throttle reference : Inport
  G Motor : TransferFcn  Numerator=[9.19]  Denominator=[0.16 1]
  Gain : Gain  Gain=2*pi/60
  Saturation : Saturate  UpperLimit=7685  LowerLimit=0
  Omega : Outport
  wires:
  G Motor/1 -> Saturation/1
  Gain/1 -> Omega/1
  Saturation/1 -> Gain/1
  Throttle reference/1 -> G Motor/1

== system SimulinkNewUpdate/Vehicle Dynamic1/actuator/Arm2/STANDARD ARM MODEL CLOCKWISE/PushPullDynamics ==
  Gamma reference : Inport
  G pushpull : TransferFcn  Numerator=[1212.73]  Denominator=[1 51.105 1212.73]
  Saturation : Saturate  UpperLimit=pi/9  LowerLimit=-pi/9
  Saturation1 : Saturate  UpperLimit=pi/9  LowerLimit=-pi/9
  Gamma : Outport
  wires:
  Gamma reference/1 -> Saturation/1
  G pushpull/1 -> Saturation1/1
  Saturation/1 -> G pushpull/1
  Saturation1/1 -> Gamma/1

== system SimulinkNewUpdate/Vehicle Dynamic1/actuator/Arm2/STANDARD ARM MODEL CLOCKWISE/ServoBlockDynamics ==
  Eta reference : Inport
  G Servoblock : TransferFcn  Numerator=[1228.05]  Denominator=[1 49.1806 1228.05]
  Saturation : Saturate  UpperLimit=pi/9  LowerLimit=-pi/9
  Saturation1 : Saturate  UpperLimit=pi/9  LowerLimit=-pi/9
  Eta : Outport
  wires:
  Eta reference/1 -> Saturation/1
  G Servoblock/1 -> Saturation1/1
  Saturation/1 -> G Servoblock/1
  Saturation1/1 -> Eta/1

== system SimulinkNewUpdate/Vehicle Dynamic1/actuator/Arm2/STANDARD ARM MODEL CLOCKWISE/Subsystem ==
  Vb : Inport
  pqr : Inport  Port=2
  Add : Sum
  Constant2 : Constant  Value=[0 L H]'
  Cross Product : matrix_library/Cross Product
  Reshape : Reshape  OutputDimensionality=Column vector (2-D)
  Vmotor : Outport
  wires:
  Vb/1 -> Reshape/1
  Constant2/1 -> Cross Product/1
  pqr/1 -> Cross Product/2
  Reshape/1 -> Add/1
  Cross Product/1 -> Add/2
  Add/1 -> Vmotor/1

== system SimulinkNewUpdate/Vehicle Dynamic1/actuator/Arm2/STANDARD ARM MODEL CLOCKWISE/Subsystem1 ==
  Eta : Inport
  Gamma : Inport  Port=2
  Fmotor : Inport  Port=3
  TurnDirection : Inport  Port=4
  Constant : Constant  Value=0
  Constant1 : Constant
  Constant3 : Constant
  Coordinate Transformation Conversion : robotcorelib/Coordinate Transformation Conversion  InputRepresentation=Euler Angles  InputEulerSequence=ZYX  ShowTrVecInputPort=on  OutputRepresentation=Rotation Matrix  OutputEulerSequence=ZYX  ShowTrVecOutputPort=on  SimulateUsing=Interpreted execution
      settings: LibrarySourceBlock=uavutilslib/Coordinate Transformation Conversion
  Gain1 : Gain  Gain=-1
  Gain2 : Gain  Gain=-1
  MatrixMultiply : Product  Multiplication=Matrix(*)
  Mux : Mux  Inputs=3
  Mux1 : Mux  Inputs=3
  Product : Product
  Fbody : Outport
  wires:
  Constant/1 -> Mux/1
  Eta/1 -> Gain1/1
  Gamma/1 -> Gain2/1
  Mux/1 -> Coordinate Transformation Conversion/1
  Constant1/1 -> Mux1/1
  TurnDirection/1 -> Mux1/2
  Constant3/1 -> Mux1/3
  Fmotor/1 -> Product/1
  Mux1/1 -> Product/2
  Coordinate Transformation Conversion/1 -> MatrixMultiply/1
  Product/1 -> MatrixMultiply/2
  MatrixMultiply/1 -> Fbody/1
  Gain2/1 -> Mux/3
  Gain1/1 -> Mux/2

== matlab function SimulinkNewUpdate/Subsystem1/MATLAB Function ==
  data: B output
function B = compute_B_matrix()
    % Tham số từ luận văn (ước lượng, cần điều chỉnh theo thực tế)
    mu = 0.013;        % Hệ số thrust
    kappa = 0.013;      % Hệ số torque
    J = 10^(-4);       % Moment quán tính (kg·m²)
    Omega = 100;        % Tốc độ quay propeller (rad/s)
    tr = 0.009;           % Rise time servo (s)
    L = 0.3;           % Chiều dài arm (m)
    H = 0.05;           % Chiều cao hub (m)
    T0 = 30.75;           % Thrust tại hover (N)


    % Ma trận B đầy đủ (4x12) cho 4 arms
    % Arm 1, 2, 3, 4 với rotation và dấu ± cho kappa
    B = zeros(4, 12);
    % Arm 1 
    B(:, 1:3) = [0, H*T0, J*Omega/tr;
                  L*mu, J*Omega/tr, -H*T0;
                  -kappa, L*T0, 0;
                  mu, 0, 0];
    % Arm 2 
    B(:, 4:6) = [0, -H*T0, J*Omega/tr;
                  -L*mu, J*Omega/tr, H*T0;
                  kappa, L*T0, 0;
                  mu, 0, 0];
    % Arm 3 
    B(:, 7:9) = [-L*mu, J*Omega/tr, H*T0;
                 0, H*T0, -J*Omega/tr;
                kappa, L*T0, 0;
                mu, 0, 0];
    % Arm 4 
    B(:, 10:12) = [L*mu, J*Omega/tr, -H*T0;
                 0, -H*T0, -J*Omega/tr;
                -kappa, L*T0, 0;
                mu, 0, 0];
end

== matlab function SimulinkNewUpdate/Subsystem1/MATLAB Function1 ==
  data: v input; u output; B input; W input
function u = weighted_pseudoinverse_allocator(v, B, W)
    % Input: v (4x1), B (4x12), W (12x12 diagonal)
    % Output: u (12x1)
    
    % Tính weighted pseudoinverse
    % Winv = inv(W); % Ma trận nghịch đảo trọng số
    u = W^(-1) * B' * ((B * W^(-1) * B')^(-1)) * v;
end

== matlab function SimulinkNewUpdate/Subsystem2/Subsystem/MATLAB Function ==
  data: phi input; m output; theta input; psi input
function m = fcn(phi,theta,psi)
    T_ItoV1 = [[cos(psi) sin(psi) 0];[-sin(psi) cos(psi) 0];[0 0 1]]; 
    T_V1toV2 = [[cos(theta) 0 -sin(theta)];[0 1 0];[sin(theta) 0 cos(theta)]];
    T_V2toB = [[1 0 0];[0 cos(phi) sin(phi)];[0 -sin(phi) cos(phi)]];
    m = T_V2toB*T_V1toV2*T_ItoV1

== matlab function SimulinkNewUpdate/Subsystem2/Subsystem/MATLAB Function1 ==
  data: Xe input; xb output; Ye input; psi input; yb output
function [xb,yb] = fcn(Xe,Ye,psi)
    m = [[cos(psi) sin(psi)];[-sin(psi) cos(psi)]]
    pos = m*[Xe;Ye]
    xb = pos(1)
    yb = pos(2)
